simulink model "TD_PITCH_COUPLED"  (R2019b)
settings: Solver=VariableStepAuto  StartTime=0.0  StopTime=10.0  RelTol=1e-3
undefined symbols (not defined in the file): Dm, Dt, F_limit_pitch, g, Jeq, k_pitch, k_yp, Mb
settings Model: Creator=lbend  LastModifiedBy=lbend

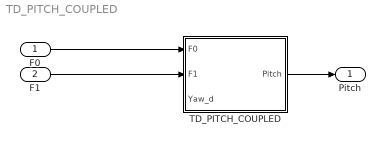
== system TD_PITCH_COUPLED ==
  F0 : Inport
  "F1 " : Inport  Port=2
  TD_PITCH_COUPLED : Subsystem
  Pitch : Outport
  wires:
  TD_PITCH_COUPLED/1(Pitch) -> Pitch/1
  F0/1 -> TD_PITCH_COUPLED/1(F0)
  "F1 "/1 -> TD_PITCH_COUPLED/2("F1 ")

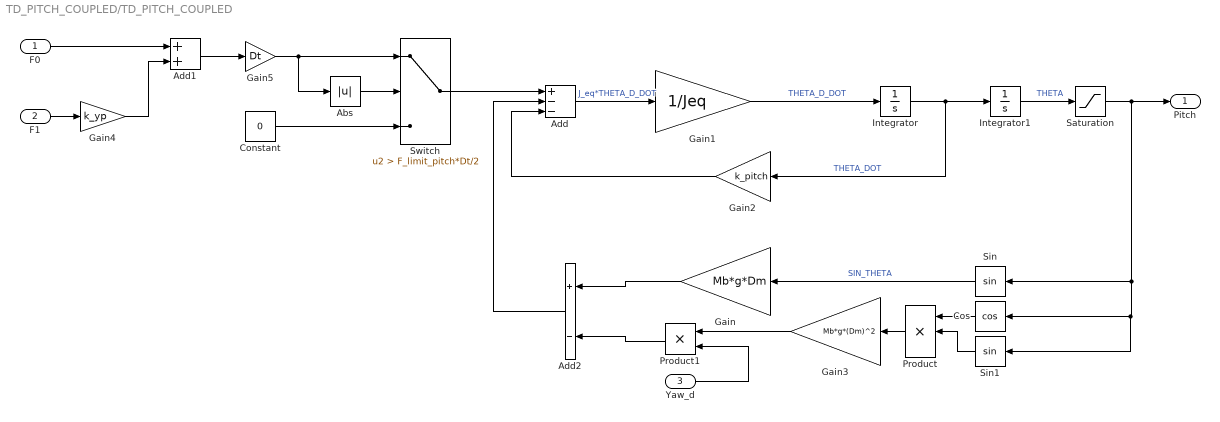
== system TD_PITCH_COUPLED/TD_PITCH_COUPLED ==
  F0 : Inport
  "F1 " : Inport  Port=2
  Yaw_d : Inport  Port=3
  Abs : Abs
  Add : Sum  Inputs=+--
  Add1 : Sum
  Add2 : Sum  Inputs=+-
  Constant : Constant  Value=0
  Cos : Trigonometry  Operator=cos
  Gain : Gain  Gain=Mb*g*Dm
  Gain1 : Gain  Gain=1/Jeq
  Gain2 : Gain  Gain=k_pitch
  Gain3 : Gain  Gain=Mb*g*(Dm)^2
  Gain4 : Gain  Gain=k_yp
  Gain5 : Gain  Gain=Dt
  Integrator : Integrator
  Integrator1 : Integrator
  Product : Product  Inputs=3
  Product1 : Product
  Saturation : Saturate  UpperLimit=0.93  LowerLimit=-0.93
  Sin : Trigonometry
  Sin1 : Trigonometry
  Switch : Switch  Criteria=u2 > Threshold  Threshold=F_limit_pitch*Dt/2
  Pitch : Outport
  wires:
  Gain2/1 -> Add/3
  Saturation/1 -> Sin1/1, Cos/1, Sin/1, Pitch/1
  Sin/1 -> Gain/1  "SIN_THETA"
  Integrator/1 -> Integrator1/1, Gain2/1  "THETA_DOT"
  Add/1 -> Gain1/1  "J_eq*THETA_D_DOT"
  Gain1/1 -> Integrator/1  "THETA_D_DOT"
  Integrator1/1 -> Saturation/1  "THETA"
  Switch/1 -> Add/1
  F0/1 -> Add1/1
  "F1 "/1 -> Gain4/1
  Gain4/1 -> Add1/2
  Gain5/1 -> Abs/1, Switch/1
  Constant/1 -> Switch/3
  Abs/1 -> Switch/2
  Add1/1 -> Gain5/1
  Sin1/1 -> Product/2
  Cos/1 -> Product/1
  Product/1 -> Gain3/1
  Gain/1 -> Add2/1
  Add2/1 -> Add/2
  Gain3/1 -> Product1/1
  Product1/1 -> Add2/2
  Yaw_d/1 -> Product1/2
